simulink model "MRAC_P1_bursting"  (R2019b)
settings: Solver=VariableStepAuto  StartTime=0.0  StopTime=17000  RelTol=1e-3
undefined symbols (not defined in the file or in its folder): sigbuilder_block
libraries: slctrlblks x5, simulink x2
settings Model: Creator=Henry  LastModifiedBy=Kevin
settings SFSimCC: CustomCodeUndefinedFunction=UseInterfaceOnly

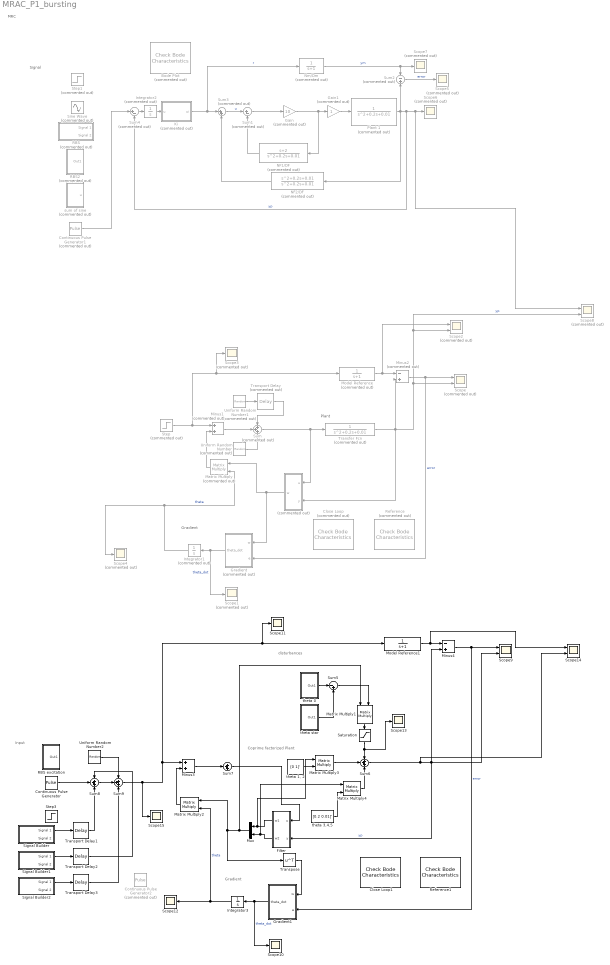
== system MRAC_P1_bursting ==
  note: Coprime factorized Plant
  note: disturbances
  note: Plant
  note: Gradient
  note: Signal
  note: MRC
  note: Gradient
  note: Input
  " " : Subsystem  Commented=on
  Bode Plot : slctrlblks/Model Verification/Check Bode  Characteristics  Commented=on  InstantiateOnLoad=on  SaveOperatingPoints=off  LinearizationIOs={'/Gain1', 1, 'in', 'off', '';'/Plant 1', 1, 'out', 'on', ''}  LinearizeAt=SnapshotTimes  SnapshotTimes=[0]  TriggerType=rising  SampleTime=auto  RateConversionMethod=zoh  PreWarpFreq=10  UseExactDelayModel=off  UseFullBlockNameLabels=off  UseBusSignalLabels=off  enabled=on  stopWhenAssertionFail=off  export=off  ViewDlgPos=[1981 -205.666666666667 1445.33333333333 714]  OpenViewOnLoad=off  LaunchViewOnOpen=off  FrequencyUnits=rad/s  MagnitudeUnits=dB  PhaseUnits=deg  TimeUnits=seconds  EnableUpperBound=off  UpperBoundFrequencies=[]  UpperBoundMagnitudes=[]  EnableLowerBound=off  LowerBoundFrequencies=[]  LowerBoundMagnitudes=[]
      settings: SourceProductName=Simulink Control Design
  Close Loop : slctrlblks/Model Verification/Check Bode  Characteristics  Commented=on  InstantiateOnLoad=on  SaveOperatingPoints=off  LinearizationIOs={'/Transfer Fcn', 1, 'out', 'off', '';'/Minus1', 1, 'in', 'off', ''}  LinearizeAt=SnapshotTimes  SnapshotTimes=[0]  TriggerType=rising  SampleTime=auto  RateConversionMethod=zoh  PreWarpFreq=10  UseExactDelayModel=off  UseFullBlockNameLabels=off  UseBusSignalLabels=off  enabled=on  stopWhenAssertionFail=off  export=off  ViewDlgPos=[100 200 510 390]  OpenViewOnLoad=off  LaunchViewOnOpen=on  FrequencyUnits=rad/s  MagnitudeUnits=dB  PhaseUnits=deg  TimeUnits=seconds  EnableUpperBound=off  UpperBoundFrequencies=[]  UpperBoundMagnitudes=[]  EnableLowerBound=off  LowerBoundFrequencies=[]  LowerBoundMagnitudes=[]
      settings: SourceProductName=Simulink Control Design
  Close Loop1 : slctrlblks/Model Verification/Check Bode  Characteristics  InstantiateOnLoad=on  SaveOperatingPoints=off  LinearizationIOs={'/Transfer Fcn', 1, 'out', 'off', '';'/Minus1', 1, 'in', 'off', ''}  LinearizeAt=SnapshotTimes  SnapshotTimes=[0]  TriggerType=rising  SampleTime=auto  RateConversionMethod=zoh  PreWarpFreq=10  UseExactDelayModel=off  UseFullBlockNameLabels=off  UseBusSignalLabels=off  enabled=on  stopWhenAssertionFail=off  export=off  ViewDlgPos=[100 200 510 390]  OpenViewOnLoad=off  LaunchViewOnOpen=on  FrequencyUnits=rad/s  MagnitudeUnits=dB  PhaseUnits=deg  TimeUnits=seconds  EnableUpperBound=off  UpperBoundFrequencies=[]  UpperBoundMagnitudes=[]  EnableLowerBound=off  LowerBoundFrequencies=[]  LowerBoundMagnitudes=[]
      settings: SourceProductName=Simulink Control Design
  Continuous Pulse Generator : DiscretePulseGenerator  PulseType=Time based  Period=60  PulseWidth=50
  Continuous Pulse Generator1 : DiscretePulseGenerator  Commented=on  PulseType=Time based  Period=1  PulseWidth=50
  Continuous Pulse Generator2 : DiscretePulseGenerator  Commented=on  PulseType=Time based  Amplitude=10  Period=1  PulseWidth=50
  Filter : Subsystem
  Gain : Gain  Commented=on  Gain=10
  Gain1 : Gain  Commented=on
  Gradient : MATLAB Function  Commented=on  TreatAsAtomicUnit=on
  Gradient1 : MATLAB Function  TreatAsAtomicUnit=on
  Integrator1 : Integrator  Commented=on
  Integrator2 : Integrator  Commented=on
  Integrator3 : Integrator
  Ki : MATLAB Function  Commented=on  TreatAsAtomicUnit=on
  Matrix Multiply : Product  Commented=on  Multiplication=Matrix(*)
  Matrix Multiply{1..4} (4 alike) : Product  Multiplication=Matrix(*)
  Minus1 : Sum  Commented=on
  Minus2 : Sum  Commented=on  Inputs=-+
  Minus3 : Sum
  Minus4 : Sum  Inputs=-+
  Model Reference : TransferFcn  Commented=on  Denominator=[1 1]
  Model Reference1 : TransferFcn  Denominator=[1 1]
  Mux : Mux  Inputs=2
  NF1/DF : TransferFcn  Commented=on  Numerator=[1 2]  Denominator=[1 0.2 0.01]
  NF2/DF : TransferFcn  Commented=on  Numerator=[1 0.2 0.01]  Denominator=[1 0.2 0.01]
  "Nm/Dm " : TransferFcn  Commented=on  Denominator=[1 1]
  Plant 1 : TransferFcn  Commented=on  Denominator=[1 ,0.2 ,0.01]
  "RBS " : Subsystem  Tag=STV Subsys  Commented=on  LoadFcn=sigbuilder_block('load');  StartFcn=sigbuilder_block('start');  StopFcn=sigbuilder_block('stop');  ClipboardFcn=sigbuilder_block('clipboard');  mask(Sigbuilder block){tuvar=[0:10]}
      mask help: Simulink:masks:SigbuilderBlock_MD
      mask init:
      | if ~strcmp(get_param(bdroot(gcbh),'SimulationStatus'),'stopped') tuvar = sigbuilder_block('maskInit'); end
      settings: CopyFcn=sigbuilder_block('copy');  DeleteFcn=sigbuilder_block('delete');  ModelCloseFcn=sigbuilder_block('modelClose');  PreSaveFcn=sigbuilder_block('preSave');  PauseFcn=sigbuilder_block('pause');  ContinueFcn=sigbuilder_block('continue');  NameChangeFcn=sigbuilder_block('namechange');  OpenFcn=sigbuilder_block('open',[215 62.5 550.5 362.5 ]);  CloseFcn=sigbuilder_block('close');
      mask Display: plot(0, 0, 100, 100,[2, 2, 32, 32, 2], [68, 8, 8, 68, 68],[32, 2], [38, 38], [32, 19, 2],[53, 60, 44], [32, 17, 17, 2],[16, 16, 31, 31]);txt = getActiveGroup(gcbh);text(2, 100, txt,'verticalAlignment', 'top');
  RBS excitation : Subsystem
  RBS2 : Subsystem  Commented=on
  Reference : slctrlblks/Model Verification/Check Bode  Characteristics  Commented=on  InstantiateOnLoad=on  SaveOperatingPoints=off  LinearizationIOs={'/Model Reference', 1, 'out', 'off', '';'/Step', 1, 'in', 'off', ''}  LinearizeAt=SnapshotTimes  SnapshotTimes=[0]  TriggerType=rising  SampleTime=auto  RateConversionMethod=zoh  PreWarpFreq=10  UseExactDelayModel=off  UseFullBlockNameLabels=off  UseBusSignalLabels=off  enabled=on  stopWhenAssertionFail=off  export=off  ViewDlgPos=[100 200 510 390]  OpenViewOnLoad=off  LaunchViewOnOpen=on  FrequencyUnits=rad/s  MagnitudeUnits=dB  PhaseUnits=deg  TimeUnits=seconds  EnableUpperBound=off  UpperBoundFrequencies=[]  UpperBoundMagnitudes=[]  EnableLowerBound=off  LowerBoundFrequencies=[]  LowerBoundMagnitudes=[]
      settings: SourceProductName=Simulink Control Design
  Reference1 : slctrlblks/Model Verification/Check Bode  Characteristics  InstantiateOnLoad=on  SaveOperatingPoints=off  LinearizationIOs={'/Model Reference', 1, 'out', 'off', '';'/Step', 1, 'in', 'off', ''}  LinearizeAt=SnapshotTimes  SnapshotTimes=[0]  TriggerType=rising  SampleTime=auto  RateConversionMethod=zoh  PreWarpFreq=10  UseExactDelayModel=off  UseFullBlockNameLabels=off  UseBusSignalLabels=off  enabled=on  stopWhenAssertionFail=off  export=off  ViewDlgPos=[100 200 510 390]  OpenViewOnLoad=off  LaunchViewOnOpen=on  FrequencyUnits=rad/s  MagnitudeUnits=dB  PhaseUnits=deg  TimeUnits=seconds  EnableUpperBound=off  UpperBoundFrequencies=[]  UpperBoundMagnitudes=[]  EnableLowerBound=off  LowerBoundFrequencies=[]  LowerBoundMagnitudes=[]
      settings: SourceProductName=Simulink Control Design
  Saturation : Saturate  UpperLimit=0.1  LowerLimit=-0.1
  Scope : Scope  Commented=on  NumInputPorts=2
  Scope{1,3..7} (6 alike) : Scope  Commented=on
  Scope{10..13,15} (5 alike) : Scope
  Scope14 : Scope  NumInputPorts=2
  Scope2 : Scope  Commented=on  NumInputPorts=2
  Scope8 : Scope  Commented=on  NumInputPorts=2
  Scope9 : Scope  NumInputPorts=2
  Signal Builder : Subsystem  Tag=STV Subsys  LoadFcn=sigbuilder_block('load');  StartFcn=sigbuilder_block('start');  StopFcn=sigbuilder_block('stop');  ClipboardFcn=sigbuilder_block('clipboard');  mask(Sigbuilder block){tuvar=[0:10]}
      mask help: Simulink:masks:SigbuilderBlock_MD
      mask init:
      | if ~strcmp(get_param(bdroot(gcbh),'SimulationStatus'),'stopped') tuvar = sigbuilder_block('maskInit'); end
      settings: CopyFcn=sigbuilder_block('copy');  DeleteFcn=sigbuilder_block('delete');  ModelCloseFcn=sigbuilder_block('modelClose');  PreSaveFcn=sigbuilder_block('preSave');  PauseFcn=sigbuilder_block('pause');  ContinueFcn=sigbuilder_block('continue');  NameChangeFcn=sigbuilder_block('namechange');  OpenFcn=sigbuilder_block('open',[1440 -240 1440 725.5 ]);  CloseFcn=sigbuilder_block('close');
      mask Display: plot(0, 0, 100, 100,[2, 2, 32, 32, 2], [68, 8, 8, 68, 68],[32, 2], [38, 38], [32, 19, 2],[53, 60, 44], [32, 17, 17, 2],[16, 16, 31, 31]);txt = getActiveGroup(gcbh);text(2, 100, txt,'verticalAlignment', 'top');
  Signal Builder1 : Subsystem  Tag=STV Subsys  LoadFcn=sigbuilder_block('load');  StartFcn=sigbuilder_block('start');  StopFcn=sigbuilder_block('stop');  ClipboardFcn=sigbuilder_block('clipboard');  mask(Sigbuilder block){tuvar=[0:10]}
      mask help: Simulink:masks:SigbuilderBlock_MD
      mask init:
      | if ~strcmp(get_param(bdroot(gcbh),'SimulationStatus'),'stopped') tuvar = sigbuilder_block('maskInit'); end
      settings: CopyFcn=sigbuilder_block('copy');  DeleteFcn=sigbuilder_block('delete');  ModelCloseFcn=sigbuilder_block('modelClose');  PreSaveFcn=sigbuilder_block('preSave');  PauseFcn=sigbuilder_block('pause');  ContinueFcn=sigbuilder_block('continue');  NameChangeFcn=sigbuilder_block('namechange');  OpenFcn=sigbuilder_block('open',[1759.5 -16 550.5 250 ]);  CloseFcn=sigbuilder_block('close');
      mask Display: plot(0, 0, 100, 100,[2, 2, 32, 32, 2], [68, 8, 8, 68, 68],[32, 2], [38, 38], [32, 19, 2],[53, 60, 44], [32, 17, 17, 2],[16, 16, 31, 31]);txt = getActiveGroup(gcbh);text(2, 100, txt,'verticalAlignment', 'top');
  Signal Builder2 : Subsystem  Tag=STV Subsys  LoadFcn=sigbuilder_block('load');  StartFcn=sigbuilder_block('start');  StopFcn=sigbuilder_block('stop');  ClipboardFcn=sigbuilder_block('clipboard');  mask(Sigbuilder block){tuvar=[0:10]}
      mask help: Simulink:masks:SigbuilderBlock_MD
      mask init:
      | if ~strcmp(get_param(bdroot(gcbh),'SimulationStatus'),'stopped') tuvar = sigbuilder_block('maskInit'); end
      settings: CopyFcn=sigbuilder_block('copy');  DeleteFcn=sigbuilder_block('delete');  ModelCloseFcn=sigbuilder_block('modelClose');  PreSaveFcn=sigbuilder_block('preSave');  PauseFcn=sigbuilder_block('pause');  ContinueFcn=sigbuilder_block('continue');  NameChangeFcn=sigbuilder_block('namechange');  OpenFcn=sigbuilder_block('open',[1759.5 -16 550.5 250 ]);  CloseFcn=sigbuilder_block('close');
      mask Display: plot(0, 0, 100, 100,[2, 2, 32, 32, 2], [68, 8, 8, 68, 68],[32, 2], [38, 38], [32, 19, 2],[53, 60, 44], [32, 17, 17, 2],[16, 16, 31, 31]);txt = getActiveGroup(gcbh);text(2, 100, txt,'verticalAlignment', 'top');
  Sine Wave : Sin  Commented=on  Frequency=0.1  SampleTime=0
  Step : Step  Commented=on  SampleTime=0
  Step1 : Step  Commented=on  SampleTime=0
  Step3 : Step  SampleTime=0
  Sum : Sum  Commented=on  Inputs=+++
  Sum1 : Sum  Commented=on  Inputs=|+-
  Sum2 : Sum  Commented=on  Inputs=-+
  Sum3 : Sum  Commented=on  Inputs=|++
  Sum4 : Sum  Commented=on  Inputs=|+-
  Sum5 : Sum  Inputs=|-+
  Sum{6..9} (4 alike) : Sum  Inputs=+++
  Transfer Fcn : TransferFcn  Commented=on  Denominator=[1 ,0.2 ,0.01]
  Transport Delay : TransportDelay  Commented=on  DelayTime=150
  Transport Delay1 : TransportDelay  DelayTime=5000
  Transport Delay2 : TransportDelay  DelayTime=10000
  Transport Delay3 : TransportDelay  DelayTime=15000
  Transpose : Math  Operator=transpose  SignedPower=off  SaturateOnIntegerOverflow=on
  Uniform Random Number : UniformRandomNumber  Commented=on  SampleTime=0.05
  Uniform Random Number1 : UniformRandomNumber  Commented=on  Minimum=-5  Maximum=5  SampleTime=0.05
  Uniform Random Number2 : UniformRandomNumber  Minimum=-0.1  Maximum=0.1  SampleTime=0.1
  sum of sine : Subsystem  Commented=on
  "theta 0 " : Subsystem
  "theta 1, 2" : Constant  Value=[0 1]'
  theta 3,4,5 : Constant  Value=[0.2 0.01]'
  theta star : Subsystem
  wires:
  Model Reference/1 -> Scope2/1, Minus2/1
  Transfer Fcn/1 -> " "/2("y "), Scope8/2, Scope2/2, Scope/2, Minus2/2  "yp"
  Step/1 -> Scope3/1, Model Reference/1, Minus1/1
  Sum/1 -> " "/1("u "), Transfer Fcn/1
  Matrix Multiply/1 -> Minus1/2
  Gradient/1(theta_dot) -> Scope1/1, Integrator1/1  "theta_dot"
  " "/1(w) -> Gradient/1(w), Matrix Multiply/1
  Minus2/1 -> Scope/1, Gradient/2(e)  "error"
  Integrator1/1 -> Matrix Multiply/2, Scope4/1  "theta"
  Uniform Random Number/1 -> Sum/3
  Minus1/1 -> Sum/2
  Uniform Random Number1/1 -> Transport Delay/1
  Transport Delay/1 -> Sum/1
  NF1/DF/1 -> Sum1/2
  NF2/DF/1 -> Sum3/2
  Sum1/1 -> Gain/1
  Gain/1 -> Gain1/1, NF1/DF/1
  Sum4/1 -> Integrator2/1
  "Nm/Dm "/1 -> Scope7/1, Sum2/1  "ym"
  Gain1/1 -> Plant 1/1
  Ki/1(ui) -> "Nm/Dm "/1, Sum3/1  "r"
  Continuous Pulse Generator1/1 -> Sum4/1
  Sum3/1 -> Sum1/1  "u"
  Integrator2/1 -> Ki/1(u)
  Plant 1/1 -> Scope8/1, Scope6/1, Sum4/2, NF2/DF/1, Sum2/2  "yp"
  Sum2/1 -> Scope5/1  "error"
  "theta 0 "/1(Out1) -> Sum5/1
  theta star/1(Out1) -> Sum5/2
  Matrix Multiply1/1 -> Saturation/1
  Saturation/1 -> Sum6/1, Scope13/1
  Matrix Multiply3/1 -> Sum6/2
  Matrix Multiply4/1 -> Sum6/3
  Integrator3/1 -> Scope12/1, Matrix Multiply2/2  "theta"
  Matrix Multiply2/1 -> Minus3/2
  Minus3/1 -> Sum7/2
  Mux/1 -> Matrix Multiply1/1, Transpose/1, Matrix Multiply2/1
  Model Reference1/1 -> Scope14/1, Minus4/1
  Gradient1/1(theta_dot) -> Scope10/1, Integrator3/1  "theta_dot"
  Minus4/1 -> Scope9/1, Gradient1/2(e)  "error"
  Sum9/1 -> Scope15/1, Scope11/1, Model Reference1/1, Minus3/1
  Sum6/1 -> Scope14/2, Filter/2("y "), Scope9/2, Minus4/2  "yp"
  Sum7/1 -> Filter/1("u ")
  Filter/1(w1) -> Matrix Multiply3/1, Mux/1
  Filter/2(w2) -> Matrix Multiply4/1, Mux/2
  "theta 1, 2"/1 -> Matrix Multiply3/2
  theta 3,4,5/1 -> Matrix Multiply4/2
  Sum5/1 -> Matrix Multiply1/2
  Transpose/1 -> Gradient1/1(w)
  Continuous Pulse Generator/1 -> Sum8/2
  Signal Builder/1(Signal 1) -> Transport Delay1/1
  Signal Builder1/1(Signal 1) -> Transport Delay2/1
  Transport Delay1/1 -> Sum8/3
  Transport Delay2/1 -> Sum8/1
  Sum8/1 -> Sum9/2
  Transport Delay3/1 -> Sum9/3
  Uniform Random Number2/1 -> Sum9/1
  Signal Builder2/1(Signal 1) -> Transport Delay3/1

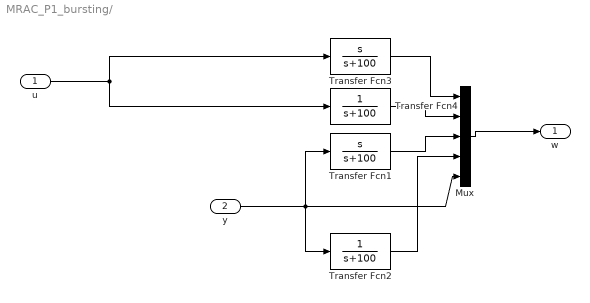
== system MRAC_P1_bursting/  ==
  "u " : Inport
  "y " : Inport  Port=2
  Mux : Mux  Inputs=5
  Transfer Fcn1 : TransferFcn  Numerator=[1 0]  Denominator=[1 100]
  Transfer Fcn2 : TransferFcn  Denominator=[1 100]
  Transfer Fcn3 : TransferFcn  Numerator=[1 0]  Denominator=[1 100]
  Transfer Fcn4 : TransferFcn  Denominator=[1 100]
  w : Outport
  wires:
  Transfer Fcn1/1 -> Mux/3
  "u "/1 -> Transfer Fcn3/1, Transfer Fcn4/1
  Mux/1 -> w/1
  "y "/1 -> Mux/5, Transfer Fcn2/1, Transfer Fcn1/1
  Transfer Fcn2/1 -> Mux/4
  Transfer Fcn3/1 -> Mux/1
  Transfer Fcn4/1 -> Mux/2

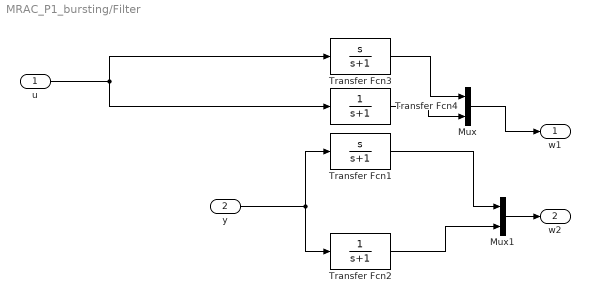
== system MRAC_P1_bursting/Filter ==
  "u " : Inport
  "y " : Inport  Port=2
  Mux : Mux  Inputs=2
  Mux1 : Mux  Inputs=2
  Transfer Fcn1 : TransferFcn  Numerator=[1 0]  Denominator=[1 1]
  Transfer Fcn2 : TransferFcn  Denominator=[1 1]
  Transfer Fcn3 : TransferFcn  Numerator=[1 0]  Denominator=[1 1]
  Transfer Fcn4 : TransferFcn  Denominator=[1 1]
  w1 : Outport
  w2 : Outport  Port=2
  wires:
  Transfer Fcn1/1 -> Mux1/1
  "u "/1 -> Transfer Fcn3/1, Transfer Fcn4/1
  Mux/1 -> w1/1
  "y "/1 -> Transfer Fcn2/1, Transfer Fcn1/1
  Transfer Fcn2/1 -> Mux1/2
  Transfer Fcn3/1 -> Mux/1
  Transfer Fcn4/1 -> Mux/2
  Mux1/1 -> w2/1

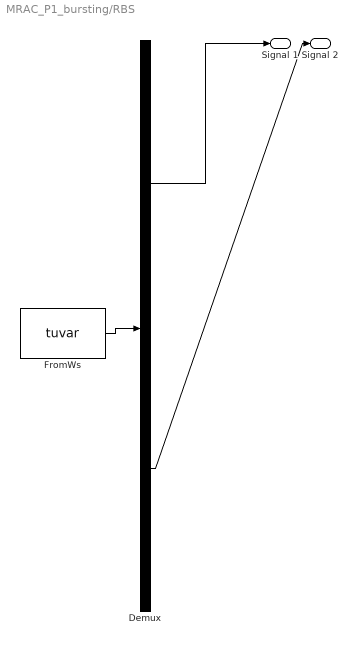
== system MRAC_P1_bursting/RBS  ==
  Demux : Demux  Tag=STV Demux  Outputs=2
  FromWs : FromWorkspace  Tag=STV FromWs  VariableName=tuvar  SampleTime=0
      SigBuilderData=|
      | common.afterFinalStr = 'Extrapolate'
      | common.sampleTime = 0
      | dataSet.timeRange = [0 10]
      | dataSet.name = 'Group 1'
      | sbobj.Groups.Name = 'Group 1'
      | sbobj.Groups.Signals(1).Name = 'Signal 1'
      | sbobj.Groups.Signals(1).XData = [0 4 4 6 6 10]
      | sbobj.Groups.Signals(1).YData = [0 0 1 1 0 0]
      | sbobj.Groups.Signals(2).Name = 'Signal 2'
      | sbobj.Groups.Signals(2).XData = [0 0.2 0.2 0.3 0.3 0.5 0.5 0.7 0.7 1 1 1.1 1.1 1.3 1.3 1.4 1.4 1.5 1.5 1.7 1.7 2.1 2.1 2.2 2.2 2.7 2.7 2.8 2.8 2.9 2.9 3 3 3.1 3.1 3.5 3.5 3.7 3.7 3.8 3.8 3.9 3.9 4.2 4.2 4.4 4.4 4.7 4.7 5 5 5.1 5.1 5.3 5.3 5.6 5.6 5.7 5.7 5.8 5.8 5.9 5.9 6 6 6.1 6.1 6.2 6.2 6.7 6.7 7 7 7.1 7.1 7.2 7.2 7.3 7.3 7.4 7.4 7.5 7.5 7.8 7.8 7.9 7.9 8.1 8.1 8.5 8.5 8.6 8.6 8.8 8.8 8.9 8.9 9 9 9.2 9.2 9.5 9.5 9.6 9.6 9.7 9.7 10]
      | sbobj.Groups.Signals(2).YData = [1 1 0 0 1 1 0 0 1 1 0 0 1 1 0 0 1 1 0 0 1 1 0 0 1 1 0 0 1 1 0 0 1 1 0 0 1 1 0 0 1 1 0 0 1 1 0 0 1 1 0 0 1 1 0 0 1 1 0 0 1 1 0 0 1 1 0 0 1 1 0 0 1 1 0 0 1 1 0 0 1 1 0 0 1 1 0 0 1 1 0 0 1 1 0 0 1 1 0 0 1 1 0 0 1 1 0 0]
  Signal 1 : Outport  Tag=STV Outport
  Signal 2 : Outport  Tag=STV Outport  Port=2
  wires:
  Demux/1 -> Signal 1/1
  FromWs/1 -> Demux/1
  Demux/2 -> Signal 2/1

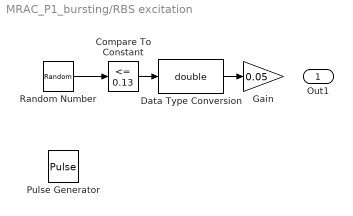
== system MRAC_P1_bursting/RBS excitation ==
  Compare To Constant : simulink/Logic and Bit Operations/Compare To Constant  relop=<=  const=0.13  OutDataTypeStr=boolean
  Data Type Conversion : DataTypeConversion  OutDataTypeStr=double
  Gain : Gain  Gain=0.05
  Pulse Generator : DiscretePulseGenerator  PulseType=Time based  Amplitude=0.01  Period=10  PulseWidth=5
  Random Number : RandomNumber  Mean=0.1  Variance=0.1  SampleTime=1
  Out1 : Outport
  wires:
  Random Number/1 -> Compare To Constant/1
  Compare To Constant/1 -> Data Type Conversion/1
  Data Type Conversion/1 -> Gain/1

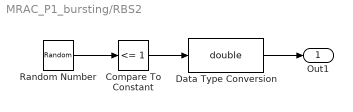
== system MRAC_P1_bursting/RBS2 ==
  Compare To Constant : simulink/Logic and Bit Operations/Compare To Constant  relop=<=  const=1  OutDataTypeStr=boolean
  Data Type Conversion : DataTypeConversion  OutDataTypeStr=double
  Random Number : RandomNumber  Mean=1  SampleTime=10
  Out1 : Outport
  wires:
  Random Number/1 -> Compare To Constant/1
  Compare To Constant/1 -> Data Type Conversion/1
  Data Type Conversion/1 -> Out1/1

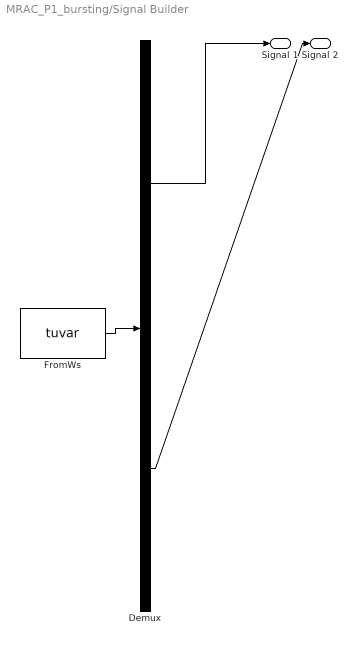
== system MRAC_P1_bursting/Signal Builder ==
  Demux : Demux  Tag=STV Demux  Outputs=2
  FromWs : FromWorkspace  Tag=STV FromWs  VariableName=tuvar  SampleTime=0
      SigBuilderData=|
      | common.afterFinalStr = 'Extrapolate'
      | common.sampleTime = 0
      | dataSet.timeRange = [0 100.6]
      | dataSet.name = 'Group 1'
      | sbobj.Groups.Name = 'Group 1'
      | sbobj.Groups.Signals(1).Name = 'Signal 1'
      | sbobj.Groups.Signals(1).XData = [0 0.5 0.5 1 1 1.5 1.5 2 2 2.5 2.5 3 3 3.5 3.5 4 4 4.5 4.5 5 5 5.5 5.5 6 6 6.5 6.5 7 7 7.5 7.5 8 8 8.5 8.5 9 9 9.5 9.5 10 10 10.5 10.5 11 11 11.5 11.5 12 12 12.5 12.5 13 13 13.5 13.5 14 14 14.5 14.5 15 15 15.5 15.5 16 16 16.5 16.5 17 17 17.5 17.5 18 18 18.5 18.5 19 19 19.5 19.5 20 20 20.5 20.5 21 21 21.5 21.5 22 22 22.5 22.5 23 23 23.5 23.5 24 24 24.5 24.5 25 25 25.5 25.5 26 26 26.5 26.5 27 27 27.5 27.5 28 28 28.5 28.5 29 29 29.5 29.5 30 30 30.5 30.5 31 31 31.5 31.5 32 32 32.5 32.5 33 33 33.5 33.5 34 34 34.5 34.5 35 35 35.5 35.5 36 36 36.5 36.5 37 37 37.5 37.5 38 38 38.5 38.5 39 39 39.5 39.5 40 40 40.5 40.5 41 41 41.5 41.5 42 42 42.5 42.5 43 43 43.5 43.5 44 44 44.5 44.5 45 45 45.5 45.5 46 46 46.5 46.5 47 47 47.5 47.5 48 48 48.5 48.5 49 49 49.5 49.5 50 50 50.5 50.5 51 51 51.5 51.5 52 52 52.5 52.5 53 53 53.5 53.5 54 54 54.5 54.5 55 55 55.5 55.5 56 56 56.5 56.5 57 57 57.5 57.5 58 58 58.5 58.5 59 59 59.5 59.5 60 60 60.5 60.5 61 61 61.5 61.5 62 62 62.5 62.5 63 63 63.5 63.5 64 64 64.5 64.5 65 65 65.5 65.5 66 66 66.5 66.5 67 67 67.5 67.5 68 68 68.5 68.5 69 69 69.5 69.5 70 70 70.5 70.5 71 71 71.5 71.5 72 72 72.5 72.5 73 73 73.5 73.5 74 74 74.5 74.5 75 75 75.5 75.5 76 76 76.5 76.5 77 77 77.5 77.5 78 78 78.5 78.5 79 79 79.5 79.5 80 80 80.5 80.5 81 81 81.5 81.5 82 82 82.5 82.5 83 83 83.5 83.5 84 84 84.5 84.5 85 85 85.5 85.5 86 86 86.5 86.5 87 87 87.5 87.5 88 88 88.5 88.5 89 89 89.5 89.5 90 90 90.5 90.5 91 91 91.5 91.5 92 92 92.5 92.5 93 93 93.5 93.5 94 94 94.5 94.5 95 95 95.5 95.5 96 96 96.5 96.5 97 97 97.5 97.5 98 98 98.5 98.5 99 99 99.5 99.5 100 100 100.5 100.5 100.6]
      | sbobj.Groups.Signals(1).YData = [20 20 0 0 20 20 0 0 20 20 0 0 20 20 0 0 20 20 0 0 20 20 0 0 20 20 0 0 20 20 0 0 20 20 0 0 20 20 0 0 20 20 0 0 20 20 0 0 20 20 0 0 20 20 0 0 20 20 0 0 20 20 0 0 20 20 0 0 20 20 0 0 20 20 0 0 20 20 0 0 20 20 0 0 20 20 0 0 20 20 0 0 20 20 0 0 20 20 0 0 20 20 0 0 20 20 0 0 20 20 0 0 20 20 0 0 20 20 0 0 20 20 0 0 20 20 0 0 20 20 0 0 20 20 0 0 20 20 0 0 20 20 0 0 20 20 0 0 20 20 0 0 20 20 0 0 20 20 0 0 20 20 0 0 20 20 0 0 20 20 0 0 20 20 0 0 20 20 0 0 20 20 0 0 20 20 0 0 20 20 0 0 20 20 0 0 20 20 0 0 20 20 0 0 20 20 0 0 20 20 0 0 20 20 0 0 20 20 0 0 20 20 0 0 20 20 0 0 20 20 0 0 20 20 0 0 20 20 0 0 20 20 0 0 20 20 0 0 20 20 0 0 20 20 0 0 20 20 0 0 20 20 0 0 20 20 0 0 20 20 0 0 20 20 0 0 20 20 0 0 20 20 0 0 20 20 0 0 20 20 0 0 20 20 0 0 20 20 0 0 20 20 0 0 20 20 0 0 20 20 0 0 20 20 0 0 20 20 0 0 20 20 0 0 20 20 0 0 20 20 0 0 20 20 0 0 20 20 0 0 20 20 0 0 20 20 0 0 20 20 0 0 20 20 0 0 20 20 0 0 20 20 0 0 20 20 0 0 20 20 0 0 20 20 0 0 20 20 0 0 20 20 0 0 20 20 0 0 20 20 0 0 20 20 0 0 20 20 0 0 20 20 0 0]
      | sbobj.Groups.Signals(2).Name = 'Signal 2'
      | sbobj.Groups.Signals(2).XData = [0 100.6]
      | sbobj.Groups.Signals(2).YData = [5 5]
      | sbobj.Groups.TimeRange = [0 100.6]
  Signal 1 : Outport  Tag=STV Outport
  Signal 2 : Outport  Tag=STV Outport  Port=2
  wires:
  Demux/1 -> Signal 1/1
  FromWs/1 -> Demux/1
  Demux/2 -> Signal 2/1

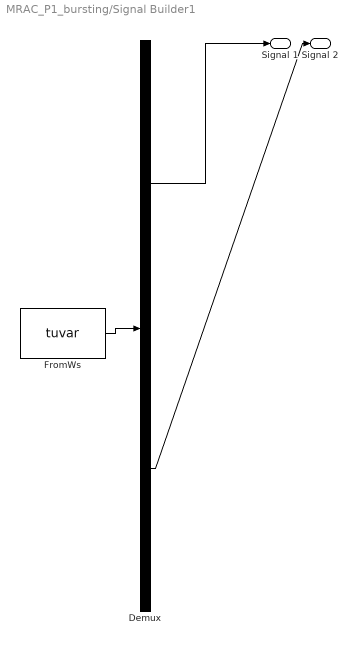
== system MRAC_P1_bursting/Signal Builder1 ==
  Demux : Demux  Tag=STV Demux  Outputs=2
  FromWs : FromWorkspace  Tag=STV FromWs  VariableName=tuvar  SampleTime=0
      SigBuilderData=|
      | common.afterFinalStr = 'Extrapolate'
      | common.sampleTime = 0
      | dataSet.timeRange = [0 100.6]
      | dataSet.name = 'Group 1'
      | sbobj.Groups.Name = 'Group 1'
      | sbobj.Groups.Signals(1).Name = 'Signal 1'
      | sbobj.Groups.Signals(1).XData = [0 0.5 0.5 1 1 1.5 1.5 2 2 2.5 2.5 3 3 3.5 3.5 4 4 4.5 4.5 5 5 5.5 5.5 6 6 6.5 6.5 7 7 7.5 7.5 8 8 8.5 8.5 9 9 9.5 9.5 10 10 10.5 10.5 11 11 11.5 11.5 12 12 12.5 12.5 13 13 13.5 13.5 14 14 14.5 14.5 15 15 15.5 15.5 16 16 16.5 16.5 17 17 17.5 17.5 18 18 18.5 18.5 19 19 19.5 19.5 20 20 20.5 20.5 21 21 21.5 21.5 22 22 22.5 22.5 23 23 23.5 23.5 24 24 24.5 24.5 25 25 25.5 25.5 26 26 26.5 26.5 27 27 27.5 27.5 28 28 28.5 28.5 29 29 29.5 29.5 30 30 30.5 30.5 31 31 31.5 31.5 32 32 32.5 32.5 33 33 33.5 33.5 34 34 34.5 34.5 35 35 35.5 35.5 36 36 36.5 36.5 37 37 37.5 37.5 38 38 38.5 38.5 39 39 39.5 39.5 40 40 40.5 40.5 41 41 41.5 41.5 42 42 42.5 42.5 43 43 43.5 43.5 44 44 44.5 44.5 45 45 45.5 45.5 46 46 46.5 46.5 47 47 47.5 47.5 48 48 48.5 48.5 49 49 49.5 49.5 50 50 50.5 50.5 51 51 51.5 51.5 52 52 52.5 52.5 53 53 53.5 53.5 54 54 54.5 54.5 55 55 55.5 55.5 56 56 56.5 56.5 57 57 57.5 57.5 58 58 58.5 58.5 59 59 59.5 59.5 60 60 60.5 60.5 61 61 61.5 61.5 62 62 62.5 62.5 63 63 63.5 63.5 64 64 64.5 64.5 65 65 65.5 65.5 66 66 66.5 66.5 67 67 67.5 67.5 68 68 68.5 68.5 69 69 69.5 69.5 70 70 70.5 70.5 71 71 71.5 71.5 72 72 72.5 72.5 73 73 73.5 73.5 74 74 74.5 74.5 75 75 75.5 75.5 76 76 76.5 76.5 77 77 77.5 77.5 78 78 78.5 78.5 79 79 79.5 79.5 80 80 80.5 80.5 81 81 81.5 81.5 82 82 82.5 82.5 83 83 83.5 83.5 84 84 84.5 84.5 85 85 85.5 85.5 86 86 86.5 86.5 87 87 87.5 87.5 88 88 88.5 88.5 89 89 89.5 89.5 90 90 90.5 90.5 91 91 91.5 91.5 92 92 92.5 92.5 93 93 93.5 93.5 94 94 94.5 94.5 95 95 95.5 95.5 96 96 96.5 96.5 97 97 97.5 97.5 98 98 98.5 98.5 99 99 99.5 99.5 100 100 100.5 100.5 100.6]
      | sbobj.Groups.Signals(1).YData = [20 20 0 0 20 20 0 0 20 20 0 0 20 20 0 0 20 20 0 0 20 20 0 0 20 20 0 0 20 20 0 0 20 20 0 0 20 20 0 0 20 20 0 0 20 20 0 0 20 20 0 0 20 20 0 0 20 20 0 0 20 20 0 0 20 20 0 0 20 20 0 0 20 20 0 0 20 20 0 0 20 20 0 0 20 20 0 0 20 20 0 0 20 20 0 0 20 20 0 0 20 20 0 0 20 20 0 0 20 20 0 0 20 20 0 0 20 20 0 0 20 20 0 0 20 20 0 0 20 20 0 0 20 20 0 0 20 20 0 0 20 20 0 0 20 20 0 0 20 20 0 0 20 20 0 0 20 20 0 0 20 20 0 0 20 20 0 0 20 20 0 0 20 20 0 0 20 20 0 0 20 20 0 0 20 20 0 0 20 20 0 0 20 20 0 0 20 20 0 0 20 20 0 0 20 20 0 0 20 20 0 0 20 20 0 0 20 20 0 0 20 20 0 0 20 20 0 0 20 20 0 0 20 20 0 0 20 20 0 0 20 20 0 0 20 20 0 0 20 20 0 0 20 20 0 0 20 20 0 0 20 20 0 0 20 20 0 0 20 20 0 0 20 20 0 0 20 20 0 0 20 20 0 0 20 20 0 0 20 20 0 0 20 20 0 0 20 20 0 0 20 20 0 0 20 20 0 0 20 20 0 0 20 20 0 0 20 20 0 0 20 20 0 0 20 20 0 0 20 20 0 0 20 20 0 0 20 20 0 0 20 20 0 0 20 20 0 0 20 20 0 0 20 20 0 0 20 20 0 0 20 20 0 0 20 20 0 0 20 20 0 0 20 20 0 0 20 20 0 0 20 20 0 0 20 20 0 0 20 20 0 0 20 20 0 0 20 20 0 0 20 20 0 0]
      | sbobj.Groups.Signals(2).Name = 'Signal 2'
      | sbobj.Groups.Signals(2).XData = [0 100.6]
      | sbobj.Groups.Signals(2).YData = [5 5]
      | sbobj.Groups.TimeRange = [0 100.6]
  Signal 1 : Outport  Tag=STV Outport
  Signal 2 : Outport  Tag=STV Outport  Port=2
  wires:
  Demux/1 -> Signal 1/1
  FromWs/1 -> Demux/1
  Demux/2 -> Signal 2/1

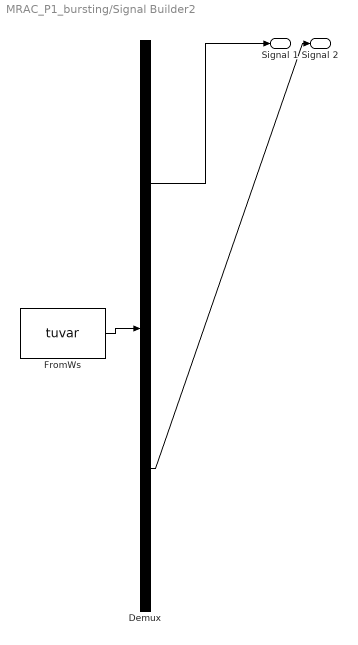
== system MRAC_P1_bursting/Signal Builder2 ==
  Demux : Demux  Tag=STV Demux  Outputs=2
  FromWs : FromWorkspace  Tag=STV FromWs  VariableName=tuvar  SampleTime=0
      SigBuilderData=|
      | common.afterFinalStr = 'Extrapolate'
      | common.sampleTime = 0
      | dataSet.timeRange = [0 100.6]
      | dataSet.name = 'Group 1'
      | sbobj.Groups.Name = 'Group 1'
      | sbobj.Groups.Signals(1).Name = 'Signal 1'
      | sbobj.Groups.Signals(1).XData = [0 0.5 0.5 1 1 1.5 1.5 2 2 2.5 2.5 3 3 3.5 3.5 4 4 4.5 4.5 5 5 5.5 5.5 6 6 6.5 6.5 7 7 7.5 7.5 8 8 8.5 8.5 9 9 9.5 9.5 10 10 10.5 10.5 11 11 11.5 11.5 12 12 12.5 12.5 13 13 13.5 13.5 14 14 14.5 14.5 15 15 15.5 15.5 16 16 16.5 16.5 17 17 17.5 17.5 18 18 18.5 18.5 19 19 19.5 19.5 20 20 20.5 20.5 21 21 21.5 21.5 22 22 22.5 22.5 23 23 23.5 23.5 24 24 24.5 24.5 25 25 25.5 25.5 26 26 26.5 26.5 27 27 27.5 27.5 28 28 28.5 28.5 29 29 29.5 29.5 30 30 30.5 30.5 31 31 31.5 31.5 32 32 32.5 32.5 33 33 33.5 33.5 34 34 34.5 34.5 35 35 35.5 35.5 36 36 36.5 36.5 37 37 37.5 37.5 38 38 38.5 38.5 39 39 39.5 39.5 40 40 40.5 40.5 41 41 41.5 41.5 42 42 42.5 42.5 43 43 43.5 43.5 44 44 44.5 44.5 45 45 45.5 45.5 46 46 46.5 46.5 47 47 47.5 47.5 48 48 48.5 48.5 49 49 49.5 49.5 50 50 50.5 50.5 51 51 51.5 51.5 52 52 52.5 52.5 53 53 53.5 53.5 54 54 54.5 54.5 55 55 55.5 55.5 56 56 56.5 56.5 57 57 57.5 57.5 58 58 58.5 58.5 59 59 59.5 59.5 60 60 60.5 60.5 61 61 61.5 61.5 62 62 62.5 62.5 63 63 63.5 63.5 64 64 64.5 64.5 65 65 65.5 65.5 66 66 66.5 66.5 67 67 67.5 67.5 68 68 68.5 68.5 69 69 69.5 69.5 70 70 70.5 70.5 71 71 71.5 71.5 72 72 72.5 72.5 73 73 73.5 73.5 74 74 74.5 74.5 75 75 75.5 75.5 76 76 76.5 76.5 77 77 77.5 77.5 78 78 78.5 78.5 79 79 79.5 79.5 80 80 80.5 80.5 81 81 81.5 81.5 82 82 82.5 82.5 83 83 83.5 83.5 84 84 84.5 84.5 85 85 85.5 85.5 86 86 86.5 86.5 87 87 87.5 87.5 88 88 88.5 88.5 89 89 89.5 89.5 90 90 90.5 90.5 91 91 91.5 91.5 92 92 92.5 92.5 93 93 93.5 93.5 94 94 94.5 94.5 95 95 95.5 95.5 96 96 96.5 96.5 97 97 97.5 97.5 98 98 98.5 98.5 99 99 99.5 99.5 100 100 100.5 100.5 100.6]
      | sbobj.Groups.Signals(1).YData = [20 20 0 0 20 20 0 0 20 20 0 0 20 20 0 0 20 20 0 0 20 20 0 0 20 20 0 0 20 20 0 0 20 20 0 0 20 20 0 0 20 20 0 0 20 20 0 0 20 20 0 0 20 20 0 0 20 20 0 0 20 20 0 0 20 20 0 0 20 20 0 0 20 20 0 0 20 20 0 0 20 20 0 0 20 20 0 0 20 20 0 0 20 20 0 0 20 20 0 0 20 20 0 0 20 20 0 0 20 20 0 0 20 20 0 0 20 20 0 0 20 20 0 0 20 20 0 0 20 20 0 0 20 20 0 0 20 20 0 0 20 20 0 0 20 20 0 0 20 20 0 0 20 20 0 0 20 20 0 0 20 20 0 0 20 20 0 0 20 20 0 0 20 20 0 0 20 20 0 0 20 20 0 0 20 20 0 0 20 20 0 0 20 20 0 0 20 20 0 0 20 20 0 0 20 20 0 0 20 20 0 0 20 20 0 0 20 20 0 0 20 20 0 0 20 20 0 0 20 20 0 0 20 20 0 0 20 20 0 0 20 20 0 0 20 20 0 0 20 20 0 0 20 20 0 0 20 20 0 0 20 20 0 0 20 20 0 0 20 20 0 0 20 20 0 0 20 20 0 0 20 20 0 0 20 20 0 0 20 20 0 0 20 20 0 0 20 20 0 0 20 20 0 0 20 20 0 0 20 20 0 0 20 20 0 0 20 20 0 0 20 20 0 0 20 20 0 0 20 20 0 0 20 20 0 0 20 20 0 0 20 20 0 0 20 20 0 0 20 20 0 0 20 20 0 0 20 20 0 0 20 20 0 0 20 20 0 0 20 20 0 0 20 20 0 0 20 20 0 0 20 20 0 0 20 20 0 0 20 20 0 0 20 20 0 0 20 20 0 0 20 20 0 0]
      | sbobj.Groups.Signals(2).Name = 'Signal 2'
      | sbobj.Groups.Signals(2).XData = [0 100.6]
      | sbobj.Groups.Signals(2).YData = [5 5]
      | sbobj.Groups.TimeRange = [0 100.6]
  Signal 1 : Outport  Tag=STV Outport
  Signal 2 : Outport  Tag=STV Outport  Port=2
  wires:
  Demux/1 -> Signal 1/1
  FromWs/1 -> Demux/1
  Demux/2 -> Signal 2/1

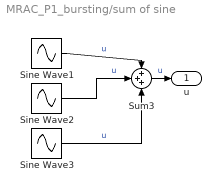
== system MRAC_P1_bursting/sum of sine ==
  Sine Wave1 : Sin  Frequency=0.1  Phase=0.1  SampleTime=0
  Sine Wave2 : Sin  SampleTime=0
  Sine Wave3 : Sin  Frequency=2  SampleTime=0
  Sum3 : Sum  Inputs=+++
  u : Outport
  wires:
  Sine Wave3/1 -> Sum3/3  "u"
  Sine Wave1/1 -> Sum3/1  "u"
  Sum3/1 -> u/1  "u"
  Sine Wave2/1 -> Sum3/2  "u"

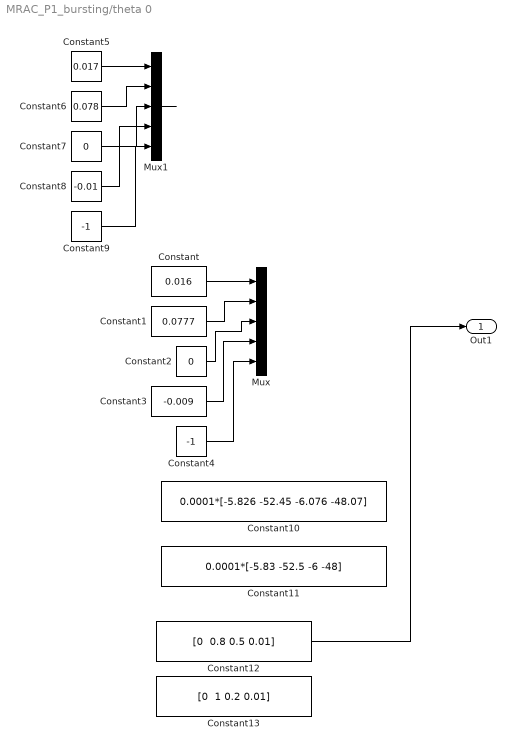
== system MRAC_P1_bursting/theta 0  ==
  Constant : Constant  Value=0.016
  Constant1 : Constant  Value=0.0777
  Constant10 : Constant  Value=0.0001*[-5.826 -52.45 -6.076 -48.07]
  Constant11 : Constant  Value=0.0001*[-5.83 -52.5 -6 -48]
  Constant12 : Constant  Value="[0  0.8 0.5 0.01]"
  Constant13 : Constant  Value="[0  1 0.2 0.01]"
  Constant2 : Constant  Value=0
  Constant3 : Constant  Value=-0.009
  Constant4 : Constant  Value=-1
  Constant5 : Constant  Value=0.017
  Constant6 : Constant  Value=0.078
  Constant7 : Constant  Value=0
  Constant8 : Constant  Value=-0.01
  Constant9 : Constant  Value=-1
  Mux : Mux  Inputs=5
  Mux1 : Mux  Inputs=5
  Out1 : Outport
  wires:
  Constant/1 -> Mux/1
  Constant3/1 -> Mux/4
  Constant2/1 -> Mux/3
  Constant4/1 -> Mux/5
  Constant1/1 -> Mux/2
  Mux1/1 -> ?
  Constant6/1 -> Mux1/2
  Constant8/1 -> Mux1/4
  Constant9/1 -> Mux1/5
  Constant7/1 -> Mux1/3
  Constant5/1 -> Mux1/1
  Constant12/1 -> Out1/1

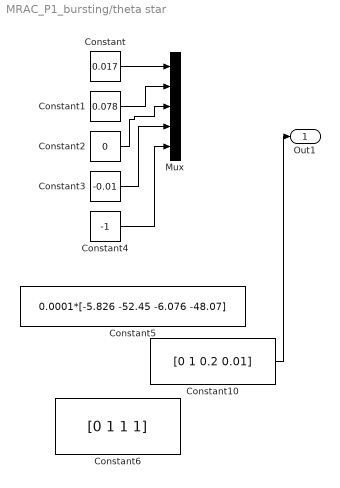
== system MRAC_P1_bursting/theta star ==
  Constant : Constant  Value=0.017
  Constant1 : Constant  Value=0.078
  Constant10 : Constant  Value=[0 1 0.2 0.01]
  Constant2 : Constant  Value=0
  Constant3 : Constant  Value=-0.01
  Constant4 : Constant  Value=-1
  Constant5 : Constant  Value=0.0001*[-5.826 -52.45 -6.076 -48.07]
  Constant6 : Constant  Value=[0 1 1 1]
  Mux : Mux  Inputs=5
  Out1 : Outport
  wires:
  Constant/1 -> Mux/1
  Constant3/1 -> Mux/4
  Constant4/1 -> Mux/5
  Constant1/1 -> Mux/2
  Constant2/1 -> Mux/3
  Constant10/1 -> Out1/1

== matlab function MRAC_P1_bursting/Gradient ==
  data: w input; theta_dot output; e input
function theta_dot = fcn(w, e)
alpha = 0.01;
I = eye(5);
gamma = alpha*I;


theta_dot = -gamma*w*e;

end

== matlab function MRAC_P1_bursting/Ki ==
  data: u input; ui output
function ui = fcn(u)
 coder.extrinsic("ss","place","matsplit",'ctrb');
% [b2, b1, b0, a1, a0] = matsplit(theta);
ui = 0;
A = [0 1; -0.01 -0.2];
B = [0 1]';
C = [1 0];

o = [0 0]';
A1 = [A o;C 0];
B1 = [B;0];
p = [-.1+0.69805i -.1-0.69805i -1];
K1 = place(A1,B1,p);
Ki = [K1(3)];
ui = Ki*u;

== matlab function MRAC_P1_bursting/Gradient1 ==
  data: w input; theta_dot output; e input
function theta_dot = fcn(w, e)
alpha = 0.05;
I = eye(4);
gamma = alpha*I;


theta_dot = -gamma*w*e;

end
